simulink library "aro"  (Simulink 8.1)
settings: Solver=ode1  StartTime=0.0  StopTime=Inf  FixedStep=0.001  RelTol=1e-3
PostLoadFcn:
  | , if any(exist('dsrtsu_mdlpostloadfcn', 'file') == [2, 3, 6]), try dsrtsu_mdlpostloadfcn('Execute', bdroot); catch fprintf('Error in PostLoadFcn (dsrtsu_mdlpostloadfcn) for model "%s":\n %s\n', bdroot, lasterr); end, end,
undefined symbols (not defined in the file or in its folder): KJUD_AEBReturnOpRelSpeedX_kph, KJUD_AEBReturnOpVehClearance_m
libraries: hcu_lib x1
settings Model: DSRTSU_INTERNAL_RTI_VER=450  DSRTSU_INTERNAL_RTI_TYPE=rti1401  RTICANMMDATA=struct('GeneralSetupData',struct('modelroot','D:\ELN150201_TAIWAN\trunk\AdasDragon\software\sw_development\arch\app\jud','generalsettings',struct('filesettings',struct('destfolder',struct('Name','RTICANMM_FILES','Check',1),'buildfolder',struct('Name','.','Check',1),'AbsDestfolder',struct('Name','D:\ELN150201_TAIWAN\trunk\AdasDragon\software\sw_development\arch\app\jud\RTICANMM_FILES'),'AbsBuildfolder',struct('Name','D:\ELN150201_TAIWAN\trunk\AdasDragon\software\sw_development\arch\app\jud'))),'options',struct('addpaths',1,'rmpaths',1,'addtrcexclusion',logical(1),'cannavigator',struct('checkmonitoring',0),'show_usrtrc',0,'use_usrtrc',0),'advanced',struct('options',[1 1 1 1 1 1 1 1 1 1 1 1 1 1 1 1 1 1 1 1 1 1 1 1 1 1 1 1 1 1 1 1 1 1 1 1 1 1 1 1 1 1 1 1 1 1 1 1 1 1 1 1 1 1 1 1 1 1 1 1 1 1 1 1 1 1 1 1 1 1 1 1 1 1 1 1 1 1 1 1 1 1 1 1 1 1 1 1 1 1 1 1 1 1 1 1 1 1 1 1]),'MPSetup',{{}},'modelname','aro','block','aro'))  DSRTSU_INTERNAL_RTIFPGA=40  Creator=AT015411  LastModifiedBy=AT015555

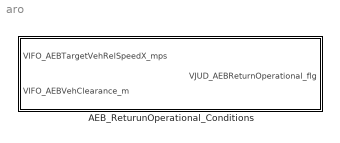
== system aro ==
  AEB_ReturunOperational_Conditions : Subsystem

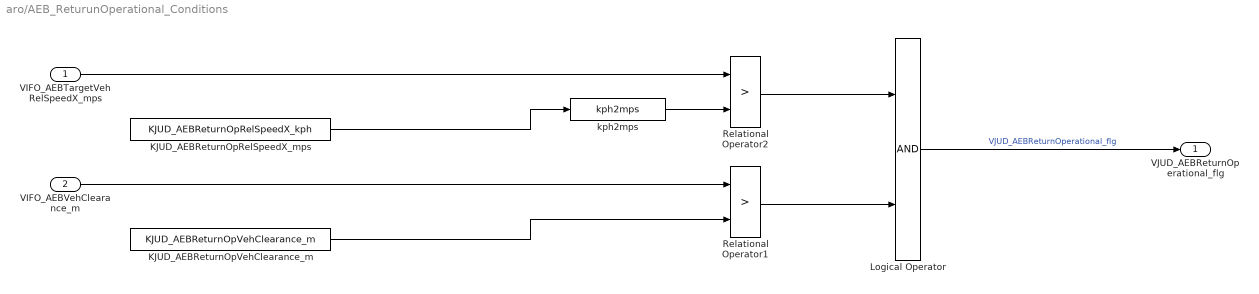
== system aro/AEB_ReturunOperational_Conditions ==
  VIFO_AEBTargetVehRelSpeedX_mps : Inport
  VIFO_AEBVehClearance_m : Inport  Port=2
  KJUD_AEBReturnOpRelSpeedX_mps : Constant  Value=KJUD_AEBReturnOpRelSpeedX_kph
  KJUD_AEBReturnOpVehClearance_m : Constant  Value=KJUD_AEBReturnOpVehClearance_m
  Logical Operator : Logic  AllPortsSameDT=off  OutDataTypeStr=boolean
  Relational Operator1 : RelationalOperator  Operator=>  OutDataTypeStr=boolean
  Relational Operator2 : RelationalOperator  Operator=>  OutDataTypeStr=boolean
  kph2mps : hcu_lib/kph2mps
  VJUD_AEBReturnOperational_flg : Outport
  wires:
  Logical Operator/1 -> VJUD_AEBReturnOperational_flg/1  "VJUD_AEBReturnOperational_flg"
  KJUD_AEBReturnOpVehClearance_m/1 -> Relational Operator1/2
  KJUD_AEBReturnOpRelSpeedX_mps/1 -> kph2mps/1
  Relational Operator1/1 -> Logical Operator/2
  Relational Operator2/1 -> Logical Operator/1
  VIFO_AEBVehClearance_m/1 -> Relational Operator1/1
  VIFO_AEBTargetVehRelSpeedX_mps/1 -> Relational Operator2/1
  kph2mps/1 -> Relational Operator2/2
